simulink model "ahu-grejac-model"  (R2021a)
settings: Solver=VariableStepAuto  StartTime=0.0  StopTime=100  RelTol=1e-3
model workspace (MATLAB code in the model file):
  | T_wo = 10;
  | T_o = 5;
  | %Twi i Tm se racunaju
  | C_ah = 4.5;              % kJ/C
  | C_pw = 4.1868;           % kJ/(kg C)
  | C_pa = 1.005;            % kJ/(kg C)
  | f_sw = 8.02e-05;         % m^3 / s
  | f_sa = 0.192;            % m^3 / s
  | Ro_a = 1.25;             % kg / m^3
  | Ro_w = 998;              % kg / m^3
  | UA_a = 0.04;             % kJ / s C
  | T_zeljeno = 22;
  | m_r = 0.12;              % kg / s
  | m_o = 0.12;              % kg / s
libraries: slpidlib x1

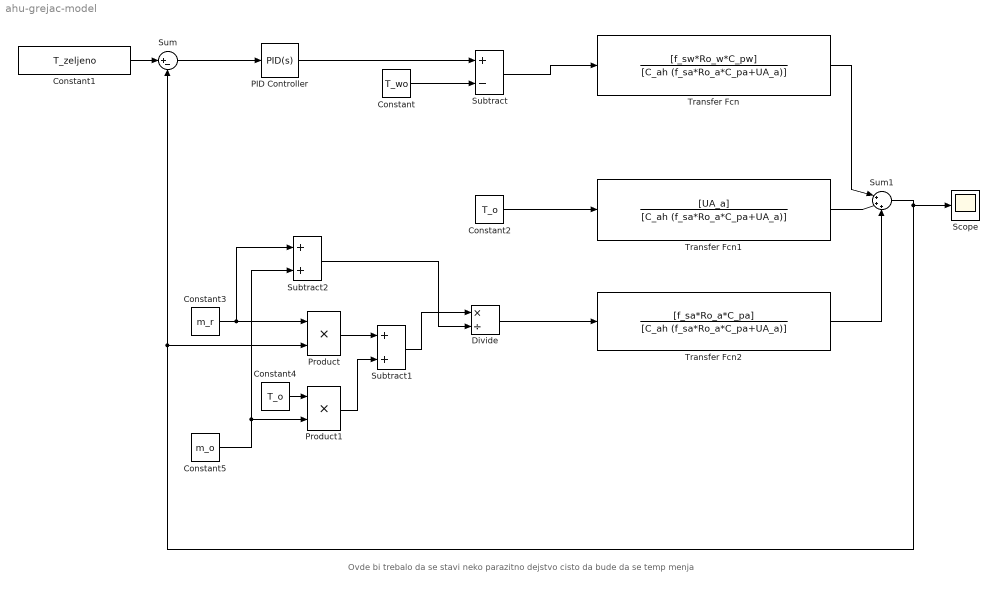
== system ahu-grejac-model ==
  note: Ovde bi trebalo da se stavi neko parazitno dejstvo cisto da bude da se temp menja
  Constant : Constant  Value=T_wo
  Constant1 : Constant  Value=T_zeljeno
  Constant2 : Constant  Value=T_o
  Constant3 : Constant  Value=m_r
  Constant4 : Constant  Value=T_o
  Constant5 : Constant  Value=m_o
  Divide : Product  Inputs=*/
  PID Controller : slpidlib/PID Controller  Controller=PID  Form=Parallel  TimeDomain=Continuous-time  UseExternalTs=off  SampleTime=-1  IntegratorMethod=Forward Euler  FilterMethod=Forward Euler  ControllerParametersSource=internal  P=15  I=1  D=0  UseFilter=on  N=100  TunerSelectOption=Transfer Function Based (PID Tuner App)  InitialConditionSource=internal  InitialConditionForIntegrator=0  InitialConditionForFilter=0  DifferentiatorICPrevScaledInput=0  ExternalReset=none  TrackingMode=off  Kt=1  LimitOutput=off  SatLimitsSource=internal  UpperSaturationLimit=inf  LowerSaturationLimit=-inf  LinearizeAsGain=on  AntiWindupMode=none  Kb=1  POutMin=[]  POutMax=[]  IOutMin=[]  IOutMax=[]  DOutMin=[]  DOutMax=[]  NOutMin=[]  NOutMax=[]  SumOutMin=[]  SumOutMax=[]  SaturationOutMin=[]  SaturationOutMax=[]  PParamMin=[]  PParamMax=[]  IParamMin=[]  IParamMax=[]  DParamMin=[]  DParamMax=[]  NParamMin=[]  NParamMax=[]  KbParamMin=[]  KbParamMax=[]  KtParamMin=[]  KtParamMax=[]  KbOutMin=[]  KbOutMax=[]  KtOutMin=[]  KtOutMax=[]  IntegratorOutMin=[]  IntegratorOutMax=[]  FilterOutMin=[]  FilterOutMax=[]  SumI1OutMin=[]  SumI1OutMax=[]  SumI2OutMin=[]  SumI2OutMax=[]  SumI3OutMin=[]  SumI3OutMax=[]  SumI4OutMin=[]  SumI4OutMax=[]  SumDOutMin=[]  SumDOutMax=[]  DifferentiatorOutMin=[]  DifferentiatorOutMax=[]  FilterDiffOutCoefMin=[]  FilterDiffOutCoefMax=[]  ReciprocalOutMin=[]  ReciprocalOutMax=[]  SumDenOutMin=[]  SumDenOutMax=[]  SumNumOutMin=[]  SumNumOutMax=[]  DivideOutMin=[]  DivideOutMax=[]  UdiffTsProdOutMin=[]  UdiffTsProdOutMax=[]  NTsProdOutMin=[]  NTsProdOutMax=[]  UintegralTsProdOutMin=[]  UintegralTsProdOutMax=[]  UngainTsProdOutMin=[]  UngainTsProdOutMax=[]  IntegratorContinuousStateAttributes=''  IntegratorStateMustResolveToSignalObject=off  IntegratorRTWStateStorageClass=Auto  FilterContinuousStateAttributes=''  FilterStateMustResolveToSignalObject=off  FilterRTWStateStorageClass=Auto  ParallelPVariant=InternalParameters  IdealPVariant=Disabled  IVariant=InternalParameters  DVariant=InternalParameters  IntegratorVariant=Continuous  SatVariant=Disabled  AWVariant=Passthrough  PCopyVariant=Disabled  TRVariant=Disabled  FdbkBlocksVariant=Forward  IdealPFdbkVariant=Disabled  SatFdbkVariant=Disabled  DerivativeFilterVariant=ContFilter  NVariant=InternalParameters  NCopyVariant=Disabled  FilterICVariant=InternalICsFilter  IntegratorICVariant=InternalICs  ExternalResetVariant=Disabled  TRSumVariant=Passthrough  SumFdbkVariant=Disabled  SumVariant=Sum_PID  TsampFilterVariant=InternalTs  TsampNgainVariant=Passthrough  TsampIntegralVariant=Passthrough  ExternalSaturationOutDataTypeStr=Inherit: Same as second input
  Product : Product
  Product1 : Product
  Scope : Scope
  Subtract : Sum  Inputs=+-
  Subtract1 : Sum
  Subtract2 : Sum
  Sum : Sum  Inputs=|+-
  Sum1 : Sum  Inputs=|+++
  Transfer Fcn : TransferFcn  Numerator=[f_sw*Ro_w*C_pw]  Denominator=[C_ah (f_sa*Ro_a*C_pa+UA_a)]
  Transfer Fcn1 : TransferFcn  Numerator=[UA_a]  Denominator=[C_ah (f_sa*Ro_a*C_pa+UA_a)]
  Transfer Fcn2 : TransferFcn  Numerator=[f_sa*Ro_a*C_pa]  Denominator=[C_ah (f_sa*Ro_a*C_pa+UA_a)]
  wires:
  Constant/1 -> Subtract/2
  Subtract/1 -> Transfer Fcn/1
  Transfer Fcn/1 -> Sum1/1
  Transfer Fcn1/1 -> Sum1/2
  Transfer Fcn2/1 -> Sum1/3
  Constant1/1 -> Sum/1
  Sum1/1 -> Scope/1, Product/2, Sum/2
  Constant2/1 -> Transfer Fcn1/1
  Constant3/1 -> Product/1, Subtract2/1
  Product/1 -> Subtract1/1
  Constant4/1 -> Product1/1
  Constant5/1 -> Product1/2, Subtract2/2
  Product1/1 -> Subtract1/2
  Subtract2/1 -> Divide/2
  Subtract1/1 -> Divide/1
  Divide/1 -> Transfer Fcn2/1
  Sum/1 -> PID Controller/1
  PID Controller/1 -> Subtract/1
